simulink model "RXsystem"  (R2024b)
settings: Solver=VariableStepAuto  StartTime=0.0  StopTime=inf  RelTol=1e-3
undefined symbols (not defined in the file or in its folder): Fs, ip, QAM, usb
libraries: commrfcorlib x3, commsync2 x2, plutoradiolib x1, commfilt2 x1, commdigbbndam3 x1
settings Model: Creator=J_mas  LastModifiedBy=J_mas

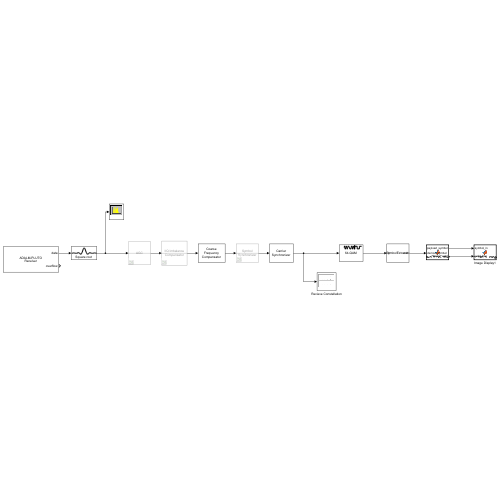
[thumbnail: Simulink's stored preview of the top-level diagram]
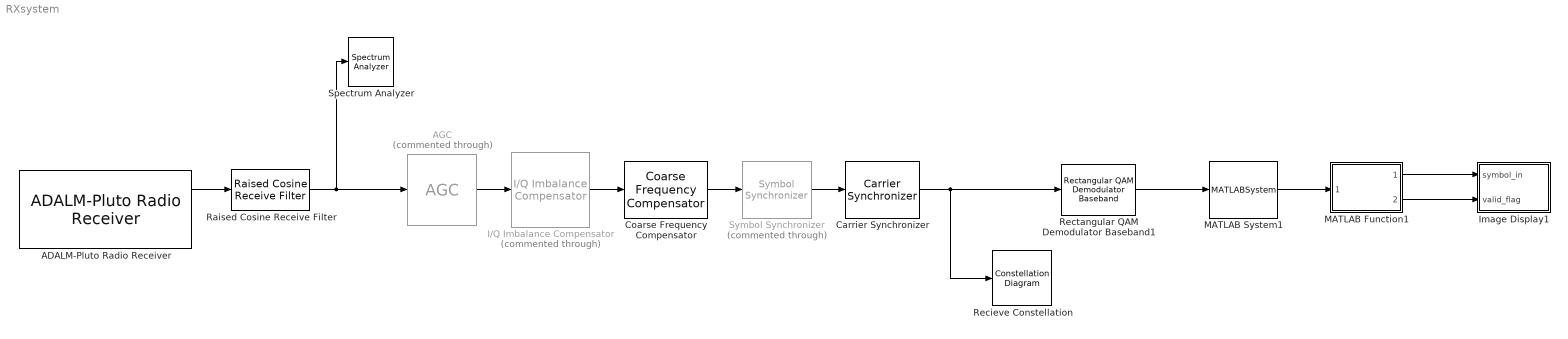
== system RXsystem ==
  ADALM-Pluto Radio Receiver : plutoradiolib/ADALM-Pluto Radio Receiver  RadioID=usb:0  uri=ip:10.0.0.200  CenterFrequencySource=Dialog  CenterFrequency=2.4e9  GainSource=AGC Slow Attack  GainSourceBlock=AGC Slow Attack  Gain=10  ChannelMapping=1  BasebandSampleRate=1e6  OutputDataType=double  SamplesPerFrame=20000  OverflowOutputPort=on  EnableBurstMode=off  NumFramesInBurst=1  ShowAdvancedProperties=off  UseCustomFilter=off  filtPathRates=[737280000 11520000 3840000 1920000 960000 240000]  filtCoefficients=[-192 82 85 -215 228 -102 -110 290 -318 145 160 -426 471 -215 -238 633 -697 318 349 -923 1009 -457 -498 1309 -1423 640 693 -1812 1959 -876 -945 2458 -2647 1180 1268 -3290 3534 -1572 -1688 4375 -4698 2091 2247 -5836 6284 -2807 -3031 7918 -8588 3870 4225 -11182 12324 -5662 -6330 17255 -19735 9507 11312 -33568 43355 -25227 -42139 305542 305542 -42139 -25227 43355 -33568 11312 9507 -19735 17255 -6330 -5662 12324 -11182 4225 3870 -8588 7918 -3031 -2807 6284 -5836 2247 2091 -4698 4375 -1688 -1572 3534 -3290 1268 1180 -2647 2458 -945 -876 1959 -1812 693 640 -1423 1309 -498 -457 1009 -923 349 318 -697 633 -238 -215 471 -426 160 145 -318 290 -110 -102 228 -215 85 82 -192]  filtCoefficientSize=128  filtDecimInterpFactor=4  filtGain=-12  filtRFBandwidth=18000000  filterConfigStruct=struct()  EnableQuadratureCorrection=on  EnableRFDCCorrection=on  EnableBasebandDCCorrection=on  FrequencyCorrection=0  OverrideSampleTime=off  SampleTime=0.02  DataTimeout=Inf  ENSMPinControlMode=None  BISTLoopbackMode=Disabled  BISTToneInject=Disabled  BISTSignalGen=PRBS  BISTToneFreq=Fs/32  BISTToneLevel=0
  AGC : commrfcorlib/AGC  Commented=through  LegacyMode=off  DetectorMethod=Rectifier  LoopMethod=Linear  UpdatePeriod=100  StepSize=0.1  AdaptationStepSize=0.01  DesiredOutputPower=1  AveragingLength=100  MaximumGain=30  MaxPowerGain=60  GainOutputPort=off  InputPowerOutputPort=off  SimulateUsing=Interpreted execution
  Carrier Synchronizer : commsync2/Carrier Synchronizer  Modulation=QAM  ModulationPhaseOffset=Auto  CustomPhaseOffset=0  SamplesPerSymbol=1  DampingFactor=1  NormalizedLoopBandwidth=0.005  EstimatedPhaseErrorOutputPort=off  SimulateUsing=Code generation
  Coarse Frequency Compensator : commrfcorlib/Coarse Frequency Compensator  Modulation=QAM  Algorithm=FFT-based  FrequencyResolution=10  MaximumFrequencyOffset=5e3  SamplesPerSymbol=4  EstimatedFreqOffsetPort=off  SimulateUsing=Code generation
      settings: LibrarySourceBlock=|
      | commsync2/Coarse Frequency
      | Compensator
  I/Q Imbalance Compensator : commrfcorlib/I//Q Imbalance Compensator  Commented=through  CoefficientSource=Estimated from input signal  InitialCoefficient=0 + 0j  StepSizeSource=Property  StepSize=0.00001  AdaptInputPort=off  CoefficientOutputPort=off  SimulateUsing=Code generation
  Image Display1 : MATLAB Function  TreatAsAtomicUnit=on
  MATLAB Function1 : MATLAB Function  TreatAsAtomicUnit=on
  MATLAB System1 : MATLABSystem  System=SymbolExtractor  SimulateUsing=Code generation
      mask Type: SymbolExtractor
      mask Display:
      | disp('SymbolExtractor');
      | port_label('input',1,'in');
      | port_label('output',1,'out');
  Raised Cosine Receive Filter : commfilt2/Raised Cosine Receive Filter  filtType=Square root  R=0.2  filtSpan=10  N=8  downFactor=8  downOffset=0  filterGain=1  InputProcessing=Columns as channels (frame based)  RateOptions=Enforce single-rate processing  framing=Mute  checkCoeff=off  variableName=rcRxFilt  currentFiltSpan=10  D=5  inputOffset=0  sampMode=Mute  saveAsFlag=0  rateMode=Downsampling  checkGain=Normalized  launchFVT=on  roundingMode=Floor  overflowMode=off  coeffDataTypeStr=Inherit: Same word length as input  coeffMin=[]  coeffMax=[]  coeffLastDataTypeStr=Inherit: Same word length as input  accumDataTypeStr=Inherit: Same as product output  accumLastDataTypeStr=Inherit: Same as product output  outputDataTypeStr=Inherit: Same as accumulator  outputMin=[]  outputMax=[]  outputLastDataTypeStr=Inherit: Same as accumulator
  Recieve Constellation : ConstellationDiagram  WindowPosition=[1152.000000,229.000000,367.000000,296.000000,]  Visible=on  ScopeFrameLocation=window  SamplesPerSymbol=8  SymbolsToDisplaySource=Property  SymbolsToDisplay=100  ReferenceConstellation=64-QAM  XLimits=[-3.19,3.19]  YLimits=[-2.54,2.54]
  Rectangular QAM Demodulator Baseband1 : commdigbbndam3/Rectangular QAM Demodulator Baseband  M=64  OutType=Integer  DecType=Hard decision  VarSource=Dialog  Variance=1  Dec=Gray  Mapping=[0:15]  PowType=Min. distance between symbols  MinDist=2  AvgPow=1  PeakPow=1  Ph=0  outDtype1=Inherit via internal rule  outDtype2=uint8  derotateFactorWordLen=16  derotateFactorDataTypeStr=Inherit: Same word length as input  derotateFactorLastDataTypeStr=Inherit: Same word length as input  denormFactorWordLen=16  denormFactorDataTypeStr=Inherit: Same word length as input  denormFactorLastDataTypeStr=Inherit: Same word length as input  prodOutWordLen=32  prodOutOverflowMode=Wrap  prodOutRoundingMode=Floor  prodOutOvFlMode=off  prodOutOvFlModeLastStrValue=off  sumWordLen=32
  Spectrum Analyzer : SpectrumAnalyzer  WindowPosition=[368.000000,230.000000,800.000000,500.000000,]  ScopeFrameLocation=window  WindowInvariantSamplesPerUpdate=on
  Symbol Synchronizer : commsync2/Symbol Synchronizer  Commented=through  Modulation=PAM/PSK/QAM  TimingErrorDetector=Gardner (non-data-aided)  SamplesPerSymbol=8  DampingFactor=1  NormalizedLoopBandwidth=0.02  DetectorGain=2.7  TimingErrorOutputPort=off  SimulateUsing=Code generation
  wires:
  ADALM-Pluto Radio Receiver/1 -> Raised Cosine Receive Filter/1
  Rectangular QAM Demodulator Baseband1/1 -> MATLAB System1/1
  AGC/1 -> I/Q Imbalance Compensator/1
  MATLAB Function1/2(frame_valid) -> Image Display1/2(valid_flag)
  Coarse Frequency Compensator/1 -> Symbol Synchronizer/1
  MATLAB Function1/1(payload_symbol) -> Image Display1/1(symbol_in)
  Symbol Synchronizer/1 -> Carrier Synchronizer/1
  MATLAB System1/1 -> MATLAB Function1/1(demod_symbol)
  Carrier Synchronizer/1 -> Recieve Constellation/1, Rectangular QAM Demodulator Baseband1/1
  I/Q Imbalance Compensator/1 -> Coarse Frequency Compensator/1
  Raised Cosine Receive Filter/1 -> Spectrum Analyzer/1, AGC/1

== matlab function RXsystem/MATLAB Function1 ==
  data: demod_symbol input size=1; payload_symbol output uint8 size=1; frame_valid output boolean size=1
function [payload_symbol, frame_valid] = barkerFrameDetector(demod_symbol)
%#codegen

% ===== Image dimensions =====
IMG_ROWS = uint32(100);
IMG_COLS = uint32(100);
PAYLOAD_LIMIT = IMG_ROWS * IMG_COLS;
% ============================

% Force fixed scalar input
sym_in = uint8(demod_symbol(1,1));

% Explicit scalar outputs
payload_symbol = uint8(0);
frame_valid    = logical(false);

persistent preambleBuffer collecting payloadCounter
if isempty(collecting)
    preambleBuffer = zeros(13,1,'uint8');
    collecting     = false;
    payloadCounter = uint32(0);
end

PREAMBLE = uint8([63;63;63;63;63;0;0;63;63;0;63;0;63]);

if ~collecting
    
    % Shift buffer
    for i = 1:12
        preambleBuffer(i) = preambleBuffer(i+1);
    end
    preambleBuffer(13) = sym_in;

    % Compare with preamble
    matches = uint8(0);
    for i = 1:13
        if preambleBuffer(i) == PREAMBLE(i)
            matches = matches + uint8(1);
        end
    end

    % Start collecting if matched
    if matches >= 11
        collecting     = true;
        payloadCounter = uint32(0);
    end

else
    
    payloadCounter = payloadCounter + 1;

    if payloadCounter <= PAYLOAD_LIMIT
        payload_symbol = sym_in;
        frame_valid    = true;
    end

    if payloadCounter >= PAYLOAD_LIMIT
        collecting     = false;
        payloadCounter = uint32(0);
    end
end

end

== matlab function RXsystem/Image Display1 ==
  data: symbol_in input; valid_flag input
function reconstruct_image(symbol_in, valid_flag) %#codegen
    coder.extrinsic('imshow', 'figure', 'drawnow', 'title');
    
    persistent imgBuffer symbolCount fig initialized IMG_ROWS IMG_COLS FRAME_LEN
    
    if isempty(initialized)
        % Define image size here OR pass as parameters if needed
        IMG_ROWS = 100;
        IMG_COLS = 100;
        
        FRAME_LEN = IMG_ROWS * IMG_COLS;
        
        imgBuffer = uint8(zeros(IMG_ROWS, IMG_COLS));
        symbolCount = 0;
        
        fig = figure('Name', 'Received Image');
        initialized = true;
    end
    
    % Only accumulate if we have valid payload data
    if valid_flag
        symbolCount = symbolCount + 1;
        
        if symbolCount <= FRAME_LEN
            imgBuffer(symbolCount) = uint8(symbol_in * 4);
        end
        
        % Display complete frame
        if symbolCount == FRAME_LEN
            imshow(imgBuffer);
            title('Received Image');
            drawnow;
            
            % Reset for next frame
            symbolCount = 0;
        end
    end
end
